simulink subsystem "ALUOpDecoder"  (R2024b)
settings: Solver=VariableStepAuto  StartTime=0.0  StopTime=10.0  RelTol=1e-3
settings Model: Creator=stefano  LastModifiedBy=stefano

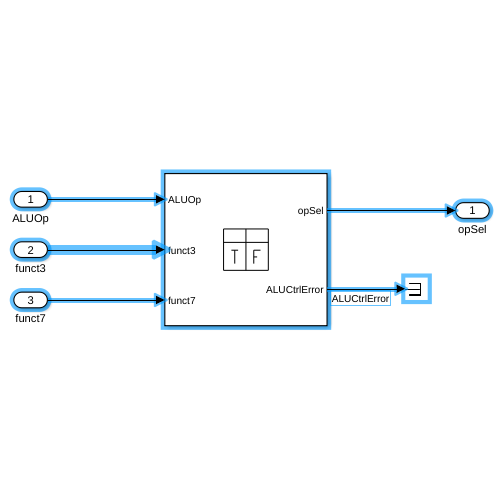
[thumbnail: Simulink's stored preview of the top-level diagram]
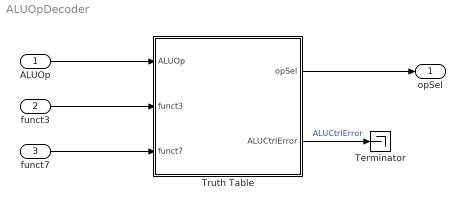
== system ALUOpDecoder ==
  ALUOp : Inport
  funct3 : Inport  Port=2
  funct7 : Inport  Port=3
  Terminator : Terminator
  Truth Table : Truth Table  TreatAsAtomicUnit=on
  opSel : Outport
  wires:
  ALUOp/1 -> Truth Table/1(ALUOp)
  Truth Table/2(ALUCtrlError) -> Terminator/1  "ALUCtrlError"
  funct7/1 -> Truth Table/3(funct7)
  Truth Table/1(opSel) -> opSel/1
  funct3/1 -> Truth Table/2(funct3)

== matlab function ALUOpDecoder/Truth Table ==
  data: ALUOp input; opSel output; funct3 input; funct7 input; ALUCtrlError output boolean
function [opSel, ALUCtrlError] = fcn(ALUOp, funct3, funct7)

aVarTruthTableCondition_1 = false;
aVarTruthTableCondition_2 = false;
aVarTruthTableCondition_3 = false;
aVarTruthTableCondition_4 = false;
aVarTruthTableCondition_5 = false;
aVarTruthTableCondition_6 = false;
aVarTruthTableCondition_7 = false;
aVarTruthTableCondition_8 = false;
aVarTruthTableCondition_9 = false;
aVarTruthTableCondition_10 = false;
aVarTruthTableCondition_11 = false;
aVarTruthTableCondition_12 = false;
aVarTruthTableCondition_13 = false;
aVarTruthTableCondition_14 = false;
aVarTruthTableCondition_15 = false;
aVarTruthTableCondition_16 = false;
aVarTruthTableCondition_17 = false;
aVarTruthTableCondition_18 = false;
aVarTruthTableCondition_19 = false;
aVarTruthTableCondition_20 = false;
aVarTruthTableCondition_21 = false;
aVarTruthTableCondition_22 = false;
aVarTruthTableCondition_23 = false;
aVarTruthTableCondition_24 = false;


% No ALU Decode

aVarTruthTableCondition_1 = logical(ALUOp == 0);

% funct3

aVarTruthTableCondition_2 = logical(ALUOp == 1);

% funct3 and funct7

aVarTruthTableCondition_3 = logical(ALUOp == 2);

% force ADD

aVarTruthTableCondition_4 = logical(ALUOp == 3);

% force SUB

aVarTruthTableCondition_5 = logical(ALUOp == 4);

% R-Type: add

aVarTruthTableCondition_6 = logical(funct7 == 0 && funct3 == 0);

% R-Type: sub

aVarTruthTableCondition_7 = logical(funct7 == 32 && funct3 == 0);

% R-Type: AND

aVarTruthTableCondition_8 = logical(funct7 == 0 && funct3 == 7);

% R-Type: OR

aVarTruthTableCondition_9 = logical(funct7 == 0 && funct3 == 6);

% R-Type: XOR

aVarTruthTableCondition_10 = logical(funct7 == 0 && funct3 == 4);

% R-Type: SLT

aVarTruthTableCondition_11 = logical(funct7 == 0 && funct3 == 2);

% R-Type: SLTU

aVarTruthTableCondition_12 = logical(funct7 == 0 && funct3 == 3);

% R-Type: SLL

aVarTruthTableCondition_13 = logical(funct7 == 0 && funct3 == 1);

% R-Type: SRL

aVarTruthTableCondition_14 = logical(funct7 == 0 && funct3 == 5);

% R-Type: SRA

aVarTruthTableCondition_15 = logical(funct7 == 32 && funct3 == 5);

% I-Type: addi

aVarTruthTableCondition_16 = logical(funct3 == 0);

% I-Type: slli

aVarTruthTableCondition_17 = logical(funct3 == 1 && funct7 == 0);

% I-Type: srli

aVarTruthTableCondition_18 = logical(funct3 == 5 && funct7 == 0);

% I-Type: srai

aVarTruthTableCondition_19 = logical(funct3 == 0 && funct7 == 32);

% I-Type: xori

aVarTruthTableCondition_20 = logical(funct3 == 4);

% I-Type: ori

aVarTruthTableCondition_21 = logical(funct3 == 6);

% I-Type: andi

aVarTruthTableCondition_22 = logical(funct3 == 7);

% I-Type: slti

aVarTruthTableCondition_23 = logical(funct3 == 2);

% I-Type: sltiu

aVarTruthTableCondition_24 = logical(funct3 == 3);

if (aVarTruthTableCondition_1 && ~aVarTruthTableCondition_2 && ~aVarTruthTableCondition_3 && ~aVarTruthTableCondition_4 && ~aVarTruthTableCondition_5)
    pt();
elseif (~aVarTruthTableCondition_1 && ~aVarTruthTableCondition_2 && ~aVarTruthTableCondition_3 && aVarTruthTableCondition_4 && ~aVarTruthTableCondition_5)
    add();
elseif (~aVarTruthTableCondition_1 && ~aVarTruthTableCondition_2 && ~aVarTruthTableCondition_3 && ~aVarTruthTableCondition_4 && aVarTruthTableCondition_5)
    sub();
elseif (~aVarTruthTableCondition_1 && ~aVarTruthTableCondition_2 && aVarTruthTableCondition_3 && ~aVarTruthTableCondition_4 && ~aVarTruthTableCondition_5 && aVarTruthTableCondition_6)
    add();
elseif (~aVarTruthTableCondition_1 && ~aVarTruthTableCondition_2 && aVarTruthTableCondition_3 && ~aVarTruthTableCondition_4 && ~aVarTruthTableCondition_5 && aVarTruthTableCondition_7)
    sub();
elseif (~aVarTruthTableCondition_1 && ~aVarTruthTableCondition_2 && aVarTruthTableCondition_3 && ~aVarTruthTableCondition_4 && ~aVarTruthTableCondition_5 && aVarTruthTableCondition_8)
    and();
elseif (~aVarTruthTableCondition_1 && ~aVarTruthTableCondition_2 && aVarTruthTableCondition_3 && ~aVarTruthTableCondition_4 && ~aVarTruthTableCondition_5 && aVarTruthTableCondition_9)
    or();
elseif (~aVarTruthTableCondition_1 && ~aVarTruthTableCondition_2 && aVarTruthTableCondition_3 && ~aVarTruthTableCondition_4 && ~aVarTruthTableCondition_5 && aVarTruthTableCondition_10)
    xor();
elseif (~aVarTruthTableCondition_1 && ~aVarTruthTableCondition_2 && aVarTruthTableCondition_3 && ~aVarTruthTableCondition_4 && ~aVarTruthTableCondition_5 && aVarTruthTableCondition_11)
    slt();
elseif (~aVarTruthTableCondition_1 && ~aVarTruthTableCondition_2 && aVarTruthTableCondition_3 && ~aVarTruthTableCondition_4 && ~aVarTruthTableCondition_5 && aVarTruthTableCondition_12)
    sltu();
elseif (~aVarTruthTableCondition_1 && ~aVarTruthTableCondition_2 && aVarTruthTableCondition_3 && ~aVarTruthTableCondition_4 && ~aVarTruthTableCondition_5 && aVarTruthTableCondition_13)
    sll();
elseif (~aVarTruthTableCondition_1 && ~aVarTruthTableCondition_2 && aVarTruthTableCondition_3 && ~aVarTruthTableCondition_4 && ~aVarTruthTableCondition_5 && aVarTruthTableCondition_14)
    srl();
elseif (~aVarTruthTableCondition_1 && ~aVarTruthTableCondition_2 && aVarTruthTableCondition_3 && ~aVarTruthTableCondition_4 && ~aVarTruthTableCondition_5 && aVarTruthTableCondition_15)
    sra();
elseif (~aVarTruthTableCondition_1 && aVarTruthTableCondition_2 && ~aVarTruthTableCondition_3 && ~aVarTruthTableCondition_4 && ~aVarTruthTableCondition_5 && aVarTruthTableCondition_16)
    add();
elseif (~aVarTruthTableCondition_1 && ~aVarTruthTableCondition_2 && aVarTruthTableCondition_3 && ~aVarTruthTableCondition_4 && ~aVarTruthTableCondition_5 && aVarTruthTableCondition_17)
    sll();
elseif (~aVarTruthTableCondition_1 && ~aVarTruthTableCondition_2 && aVarTruthTableCondition_3 && ~aVarTruthTableCondition_4 && ~aVarTruthTableCondition_5 && aVarTruthTableCondition_18)
    srl();
elseif (~aVarTruthTableCondition_1 && ~aVarTruthTableCondition_2 && aVarTruthTableCondition_3 && ~aVarTruthTableCondition_4 && ~aVarTruthTableCondition_5 && aVarTruthTableCondition_19)
    sra();
elseif (~aVarTruthTableCondition_1 && aVarTruthTableCondition_2 && ~aVarTruthTableCondition_3 && ~aVarTruthTableCondition_4 && ~aVarTruthTableCondition_5 && aVarTruthTableCondition_20)
    xor();
elseif (~aVarTruthTableCondition_1 && aVarTruthTableCondition_2 && ~aVarTruthTableCondition_3 && ~aVarTruthTableCondition_4 && ~aVarTruthTableCondition_5 && aVarTruthTableCondition_21)
    or();
elseif (~aVarTruthTableCondition_1 && aVarTruthTableCondition_2 && ~aVarTruthTableCondition_3 && ~aVarTruthTableCondition_4 && ~aVarTruthTableCondition_5 && aVarTruthTableCondition_22)
    pt();
elseif (~aVarTruthTableCondition_1 && aVarTruthTableCondition_2 && ~aVarTruthTableCondition_3 && ~aVarTruthTableCondition_4 && ~aVarTruthTableCondition_5 && aVarTruthTableCondition_23)
    slt();
elseif (~aVarTruthTableCondition_1 && aVarTruthTableCondition_2 && ~aVarTruthTableCondition_3 && ~aVarTruthTableCondition_4 && ~aVarTruthTableCondition_5 && aVarTruthTableCondition_24)
    sltu();
else % Default
    DA();
end

function DA()

% default action (should never reach)

ALUCtrlError = true;
opSel = 15;

function pt()

% passthrough

opSel = 0;
ALUCtrlError = false;

function and()

% and

opSel = 1;
ALUCtrlError = false;

function or()

% or

opSel = 2;
ALUCtrlError = false;

function add()

% add

opSel = 3;
ALUCtrlError = false;

function sub()

% sub

opSel = 4;
ALUCtrlError = false;

function slt()

% slt

opSel = 5;
ALUCtrlError = false;

function sll()

% sll

opSel = 6;
ALUCtrlError = false;

function srl()

% srl

opSel = 7;
ALUCtrlError = false;

function sra()

% sra

opSel = 8;
ALUCtrlError = false;

function xor()

% xor

opSel = 9;
ALUCtrlError = false;

function sltu()

% slt

opSel = 10;
ALUCtrlError = false;
